simulink model "StarshotACS"  (R2017a)
settings: Solver=FixedStepAuto  StartTime=0.0  StopTime=6000  FixedStep=.1  MaxStep=4.0  MinStep=.001  RelTol=1e-6
undefined symbols (not defined in the file or in its folder): DiscIntNeverNeededParam, starshot
libraries: simulink x2, dspmathops x1
settings Model: Creator=armen  LastModifiedBy=armen
settings OptimizationCC: DefaultParameterBehavior=Inlined  UseDivisionForNetSlopeComputation=on  UseFloatMulNetSlope=on  InlineInvariantSignals=on  PassReuseOutputArgsAs=Individual arguments  ZeroExternalMemoryAtStartup=off  ZeroInternalMemoryAtStartup=off  NoFixptDivByZeroProtection=on  EfficientFloat2IntCast=on  LifeSpan=1
settings DebuggingCC: ParameterTunabilityLossMsg=error  FrameProcessingCompatibilityMsg=none
settings HardwareCC: ProdBitPerPointer=32  ProdBitPerSizeT=32  ProdBitPerPtrDiffT=32  ProdLargestAtomicInteger=Long  ProdLargestAtomicFloat=Double  ProdWordSize=32  ProdHWDeviceType=ARM Compatible->ARM Cortex
settings SFSimCC: MATLABDynamicMemAlloc=off
settings RTWCC: SystemTargetFile=ert.tlc  TLCOptions=-aAlwaysIncludeCustomSrc=1  GenCodeOnly=on  TemplateMakefile=ert_default_tmf  Description=Embedded Coder  GenerateReport=on  IncludeHyperlinkInReport=on  LaunchReport=on  TargetLang=C++  GenerateTraceInfo=on  GenerateTraceReport=on  GenerateTraceReportSl=on  GenerateTraceReportSf=on  GenerateTraceReportEml=on
settings CodeAppCC: ForceParamTrailComments=on  IgnoreCustomStorageClasses=off  OperatorAnnotations=on  SimulinkDataObjDesc=on  SFDataObjDesc=on  MATLABFcnDesc=on  CustomSymbolStrGlobalVar=rt$N$M  CustomSymbolStrType=$N$M  CustomSymbolStrFcn=$N$M$F  CustomSymbolStrMacro=$N$M  InsertBlockDesc=on  MATLABSourceComments=on
settings ERTTargetCC: TargetLangStandard=C++03 (ISO)  GenerateSampleERTMain=on  IncludeMdlTerminateFcn=off  CombineSignalStateStructs=on  SupportAbsoluteTime=off  MultiInstanceERTCode=on  CodeInterfacePackaging=C++ class  SupportComplex=off  SupportNonInlinedSFcns=on  InlinedParameterPlacement=NonHierarchical  RootIOFormat=Structure reference  ERTCustomFileTemplate=example_file_process.tlc  ERTFilePackagingFormat=CompactWithDataFile

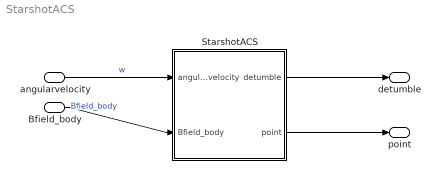
== system StarshotACS ==
  angularvelocity : Inport  OutDataTypeStr=double  PortDimensions=3  SampleTime=[0.10000000000000001 0]  Interpolate=off
  Bfield_body : Inport  Port=2  OutDataTypeStr=double  PortDimensions=3  SampleTime=[0.10000000000000001 0]  Interpolate=off
  StarshotACS : Subsystem  Tag=starshotsimv5  TreatAsAtomicUnit=on
      settings: RTWSystemCode=Inline
  detumble : Outport  OutDataTypeStr=double  PortDimensions=3  SampleTime=[0.10000000000000001 0]
  point : Outport  Port=2  OutDataTypeStr=double  PortDimensions=3  SampleTime=[0.10000000000000001 0]
  wires:
  angularvelocity/1 -> StarshotACS/1(angularvelocity)  "w"
  Bfield_body/1 -> StarshotACS/2(Bfield_body)  "Bfield_body"
  StarshotACS/1(detumble) -> detumble/1
  StarshotACS/2(point) -> point/1

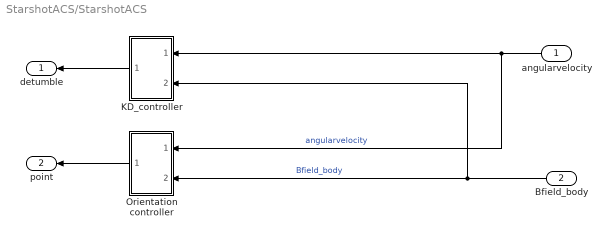
== system StarshotACS/StarshotACS ==
  angularvelocity : Inport
  Bfield_body : Inport  Port=2
  KD_controller : Subsystem
  Orientation controller : Subsystem
  detumble : Outport
  point : Outport  Port=2
  wires:
  angularvelocity/1 -> KD_controller/1(Omega), Orientation controller/1(Omega)  "angularvelocity"
  Bfield_body/1 -> Orientation controller/2(B(body)), KD_controller/2(B(body))  "Bfield_body"
  Orientation controller/1(Dipole) -> point/1
  KD_controller/1(Dipole) -> detumble/1

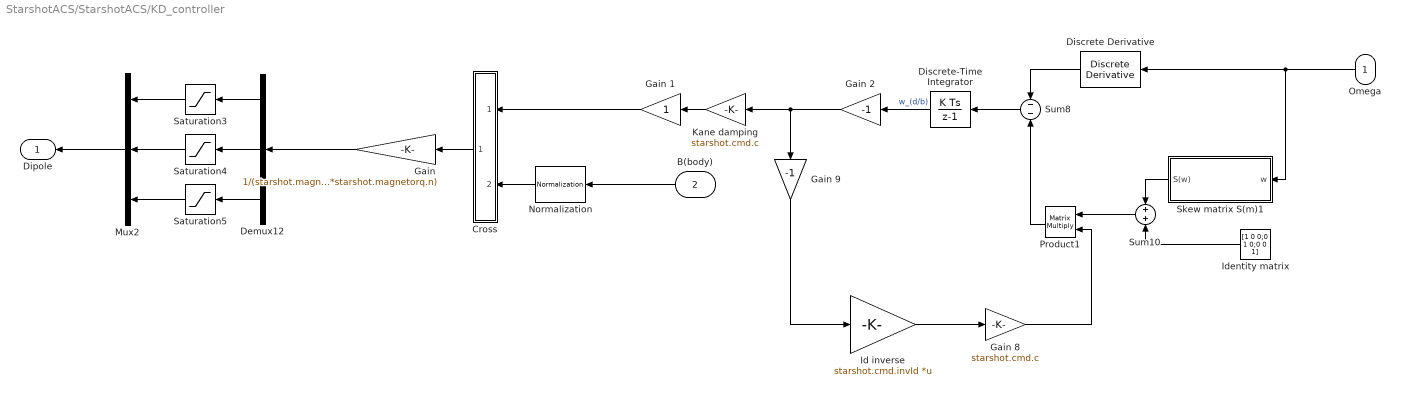
== system StarshotACS/StarshotACS/KD_controller ==
  Omega : Inport
  B(body) : Inport  Port=2
  Cross : Subsystem
  Demux12 : Demux  Outputs=3
  Discrete Derivative : simulink/Discrete/Discrete Derivative  gainval=1.0  ICPrevScaledInput=0.0  OutMin=[]  OutMax=[]  OutDataType=fixdt(1, 16)  OutScaling=2^-10  DoSatur=off
  Discrete-Time Integrator : DiscreteIntegrator  InitialCondition=starshot.cmd.wdb0  InitialConditionSetting=State (most efficient)  SampleTime=-1  ICPrevOutput=DiscIntNeverNeededParam  ICPrevScaledInput=DiscIntNeverNeededParam
  Gain : Gain  Gain=1/(starshot.magnetorq.A*starshot.magnetorq.n)
  Gain 1 : Gain  SaturateOnIntegerOverflow=on  OutDataTypeStr=Inherit: Same as input  ParamDataTypeStr=Inherit: Same as input
  Gain 2 : Gain  Gain=-1  SaturateOnIntegerOverflow=on  OutDataTypeStr=Inherit: Same as input  ParamDataTypeStr=Inherit: Same as input
  Gain 8 : Gain  Gain=starshot.cmd.c  SaturateOnIntegerOverflow=on  OutDataTypeStr=Inherit: Same as input  ParamDataTypeStr=Inherit: Same as input
  Gain 9 : Gain  Gain=-1  SaturateOnIntegerOverflow=on  OutDataTypeStr=Inherit: Same as input  ParamDataTypeStr=Inherit: Same as input
  Id inverse : Gain  Gain=starshot.cmd.invId  Multiplication=Matrix(K*u)  SaturateOnIntegerOverflow=on  OutDataTypeStr=Inherit: Same as input  ParamDataTypeStr=Inherit: Same as input
  Identity matrix : Constant  Value=[1 0 0;0 1 0;0 0 1]
  Kane damping : Gain  Gain=starshot.cmd.c  SaturateOnIntegerOverflow=on  OutDataTypeStr=Inherit: Same as input  ParamDataTypeStr=Inherit: Same as input
  Mux2 : Mux  Inputs=3
  Normalization : dspmathops/Normalization  NormType=Squared 2-norm  Bias=1e-10  NormOver=Each column  Dimension=1  outputDataTypeStr=Inherit: Same as product output  outputLastDataTypeStr=Inherit: Same as product output  outputMin=[]  outputMax=[]  accumDataTypeStr=Inherit: Same as product output  accumLastDataTypeStr=Inherit: Same as product output  roundingMode=Floor  overflowMode=off
      settings: SourceProductName=DSP System Toolbox
  Product1 : Product  Multiplication=Matrix(*)
  Saturation3 : Saturate  UpperLimit=starshot.magnetorq.m_max_x/(starshot.magnetorq.A*starshot.magnetorq.n)  LowerLimit=-starshot.magnetorq.m_max_x/(starshot.magnetorq.A*starshot.magnetorq.n)
  Saturation4 : Saturate  UpperLimit=starshot.magnetorq.m_max_y/(starshot.magnetorq.A*starshot.magnetorq.n)  LowerLimit=-starshot.magnetorq.m_max_y/(starshot.magnetorq.A*starshot.magnetorq.n)
  Saturation5 : Saturate  UpperLimit=starshot.magnetorq.m_max_z/(starshot.magnetorq.A*starshot.magnetorq.n)  LowerLimit=-starshot.magnetorq.m_max_z/(starshot.magnetorq.A*starshot.magnetorq.n)
  Skew matrix S(m)1 : Subsystem
  Sum10 : Sum  Inputs=+|+  SaturateOnIntegerOverflow=on  InputSameDT=on  OutDataTypeStr=Inherit: Same as first input
  Sum8 : Sum  Inputs=--
  Dipole : Outport
  wires:
  Mux2/1 -> Dipole/1
  Demux12/3 -> Saturation5/1
  Saturation4/1 -> Mux2/2
  Demux12/2 -> Saturation4/1
  Saturation5/1 -> Mux2/3
  Saturation3/1 -> Mux2/1
  Demux12/1 -> Saturation3/1
  Gain/1 -> Demux12/1
  Gain 1/1 -> Cross/1(A)
  Product1/1 -> Sum8/2
  Sum10/1 -> Product1/1
  Gain 9/1 -> Id inverse/1
  Identity matrix/1 -> Sum10/2
  Skew matrix S(m)1/1(S(w)) -> Sum10/1
  Id inverse/1 -> Gain 8/1
  Gain 8/1 -> Product1/2
  Sum8/1 -> Discrete-Time Integrator/1
  Discrete Derivative/1 -> Sum8/1
  Kane damping/1 -> Gain 1/1
  Normalization/1 -> Cross/2(B)
  Gain 2/1 -> Gain 9/1, Kane damping/1
  Cross/1(AxB) -> Gain/1
  B(body)/1 -> Normalization/1
  Omega/1 -> Skew matrix S(m)1/1(w), Discrete Derivative/1
  Discrete-Time Integrator/1 -> Gain 2/1  "w_(d/b)"

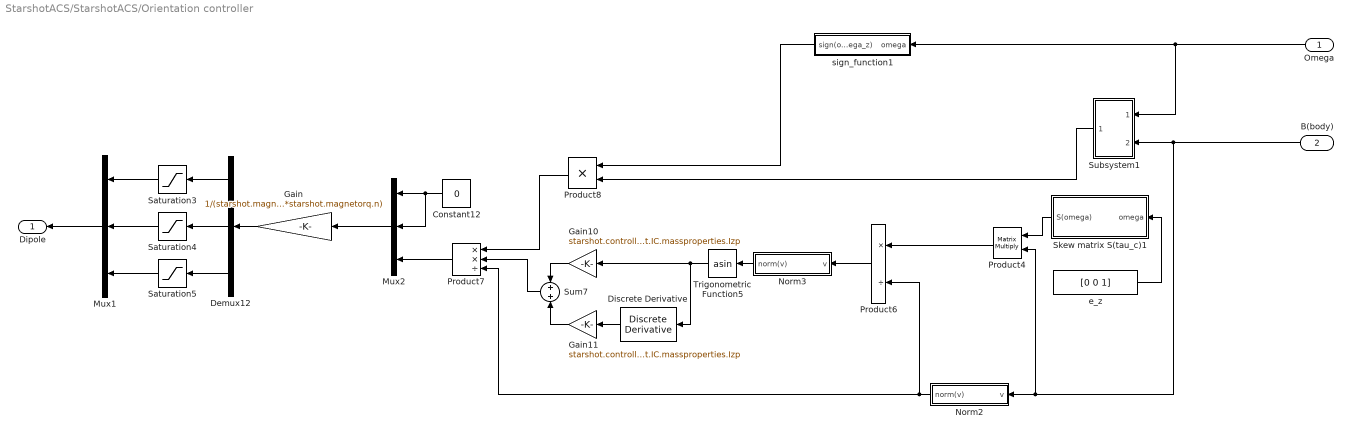
== system StarshotACS/StarshotACS/Orientation controller ==
  Omega : Inport
  B(body) : Inport  Port=2
  Constant12 : Constant  Value=0
  Demux12 : Demux  Outputs=3
  Discrete Derivative : simulink/Discrete/Discrete Derivative  gainval=1.0  ICPrevScaledInput=0.0  OutMin=[]  OutMax=[]  OutDataType=fixdt(1, 16)  OutScaling=2^-10  DoSatur=off
  Gain : Gain  Gain=1/(starshot.magnetorq.A*starshot.magnetorq.n)
  Gain10 : Gain  Gain=starshot.controller.Kp*starshot.IC.massproperties.Izp
  Gain11 : Gain  Gain=starshot.controller.Kd*starshot.IC.massproperties.Izp
  Mux1 : Mux  Inputs=3
  Mux2 : Mux  Inputs=3
  Norm2 : Subsystem
  Norm3 : Subsystem
  Product4 : Product  Multiplication=Matrix(*)
  Product6 : Product  Inputs=*/
  Product7 : Product  Inputs=**/
  Product8 : Product  Inputs=**
  Saturation3 : Saturate  UpperLimit=starshot.magnetorq.m_max_x/(starshot.magnetorq.A*starshot.magnetorq.n)  LowerLimit=-starshot.magnetorq.m_max_x/(starshot.magnetorq.A*starshot.magnetorq.n)
  Saturation4 : Saturate  UpperLimit=starshot.magnetorq.m_max_y/(starshot.magnetorq.A*starshot.magnetorq.n)  LowerLimit=-starshot.magnetorq.m_max_y/(starshot.magnetorq.A*starshot.magnetorq.n)
  Saturation5 : Saturate  UpperLimit=starshot.magnetorq.m_max_z/(starshot.magnetorq.A*starshot.magnetorq.n)  LowerLimit=-starshot.magnetorq.m_max_z/(starshot.magnetorq.A*starshot.magnetorq.n)
  Skew matrix S(tau_c)1 : Subsystem
  Subsystem1 : Subsystem
  Sum7 : Sum  Inputs=+|+
  Trigonometric Function5 : Trigonometry  Operator=asin
  e_z : Constant  Value=[0 0 1]
  sign_function1 : Subsystem
  Dipole : Outport
  wires:
  Mux1/1 -> Dipole/1
  Demux12/3 -> Saturation5/1
  Saturation4/1 -> Mux1/2
  Demux12/2 -> Saturation4/1
  Saturation5/1 -> Mux1/3
  Saturation3/1 -> Mux1/1
  Demux12/1 -> Saturation3/1
  Gain/1 -> Demux12/1
  Omega/1 -> sign_function1/1(omega), Subsystem1/1(omega)
  Subsystem1/1(sign(cos)) -> Product8/2
  sign_function1/1(sign(omega_z)) -> Product8/1
  B(body)/1 -> Subsystem1/2(B(body)), Norm2/1(v), Product4/2
  Gain11/1 -> Sum7/2
  Product8/1 -> Product7/1
  Product6/1 -> Norm3/1(v)
  Gain10/1 -> Sum7/1
  Norm2/1(norm(v)) -> Product6/2, Product7/3
  Discrete Derivative/1 -> Gain11/1
  Skew matrix S(tau_c)1/1(S(omega)) -> Product4/1
  Constant12/1 -> Mux2/1, Mux2/2
  Product7/1 -> Mux2/3
  e_z/1 -> Skew matrix S(tau_c)1/1(omega)
  Norm3/1(norm(v)) -> Trigonometric Function5/1
  Trigonometric Function5/1 -> Discrete Derivative/1, Gain10/1
  Sum7/1 -> Product7/2
  Mux2/1 -> Gain/1
  Product4/1 -> Product6/1

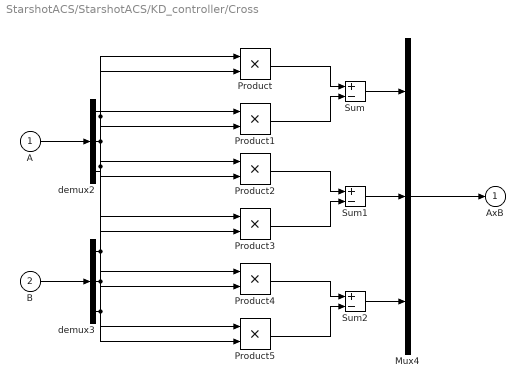
== system StarshotACS/StarshotACS/KD_controller/Cross ==
  A : Inport
  B : Inport  Port=2
  Mux4 : Mux  Inputs=3
  Product{,1..5} (6 alike) : Product  SaturateOnIntegerOverflow=on  InputSameDT=on  OutDataTypeStr=Inherit: Same as first input
  Sum : Sum  Inputs=+-  SaturateOnIntegerOverflow=on  InputSameDT=on  OutDataTypeStr=Inherit: Same as first input
  Sum1 : Sum  Inputs=+-  SaturateOnIntegerOverflow=on  InputSameDT=on  OutDataTypeStr=Inherit: Same as first input
  Sum2 : Sum  Inputs=+-  SaturateOnIntegerOverflow=on  InputSameDT=on  OutDataTypeStr=Inherit: Same as first input
  demux2 : Demux  Outputs=3
  demux3 : Demux  Outputs=3
  AxB : Outport  InitialOutput=0
  wires:
  Mux4/1 -> AxB/1
  Sum2/1 -> Mux4/3
  Sum1/1 -> Mux4/2
  Sum/1 -> Mux4/1
  Product5/1 -> Sum2/2
  Product4/1 -> Sum2/1
  Product3/1 -> Sum1/2
  Product2/1 -> Sum1/1
  Product1/1 -> Sum/2
  Product/1 -> Sum/1
  demux3/1 -> Product5/2, Product2/2
  demux2/2 -> Product5/1, Product/1
  demux3/2 -> Product4/2, Product1/2
  demux2/1 -> Product4/1, Product3/1
  demux3/3 -> Product3/2, Product/2
  demux2/3 -> Product2/1, Product1/1
  B/1 -> demux3/1
  A/1 -> demux2/1

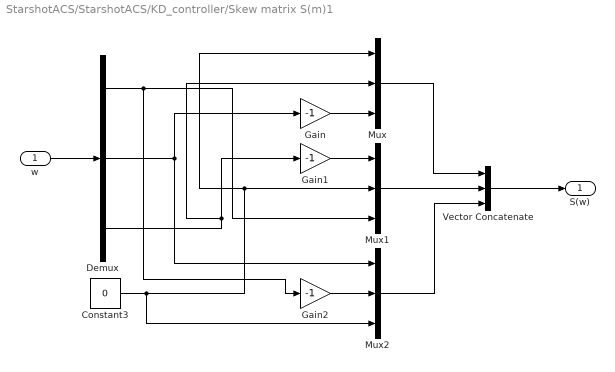
== system StarshotACS/StarshotACS/KD_controller/Skew matrix S(m)1 ==
  w : Inport
  Constant3 : Constant  Value=0
  Demux : Demux  Outputs=3
  Gain : Gain  Gain=-1
  Gain1 : Gain  Gain=-1
  Gain2 : Gain  Gain=-1
  Mux : Mux  Inputs=3
  Mux1 : Mux  Inputs=3
  Mux2 : Mux  Inputs=3
  Vector Concatenate : Concatenate  NumInputs=3  Mode=Multidimensional array  ConcatenateDimension=2
  S(w) : Outport
  wires:
  Gain1/1 -> Mux1/1
  Mux2/1 -> Vector Concatenate/3
  Mux/1 -> Vector Concatenate/1
  Vector Concatenate/1 -> S(w)/1
  Constant3/1 -> Mux1/2, Mux/1, Mux2/3
  w/1 -> Demux/1
  Mux1/1 -> Vector Concatenate/2
  Demux/1 -> Gain2/1, Mux1/3
  Gain2/1 -> Mux2/2
  Demux/3 -> Mux/2, Gain1/1
  Demux/2 -> Gain/1, Mux2/1
  Gain/1 -> Mux/3

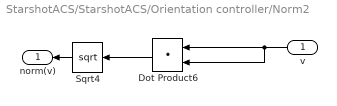
== system StarshotACS/StarshotACS/Orientation controller/Norm2 ==
  v : Inport
  Dot Product6 : DotProduct  InputSameDT=on  OutDataTypeStr=Inherit: Inherit via internal rule
  Sqrt4 : Sqrt  SaturateOnIntegerOverflow=on
  norm(v) : Outport
  wires:
  Sqrt4/1 -> norm(v)/1
  Dot Product6/1 -> Sqrt4/1
  v/1 -> Dot Product6/2, Dot Product6/1

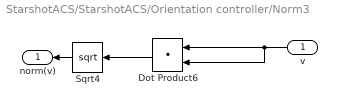
== system StarshotACS/StarshotACS/Orientation controller/Norm3 ==
  v : Inport
  Dot Product6 : DotProduct  InputSameDT=on  OutDataTypeStr=Inherit: Inherit via internal rule
  Sqrt4 : Sqrt  SaturateOnIntegerOverflow=on
  norm(v) : Outport
  wires:
  Sqrt4/1 -> norm(v)/1
  Dot Product6/1 -> Sqrt4/1
  v/1 -> Dot Product6/2, Dot Product6/1

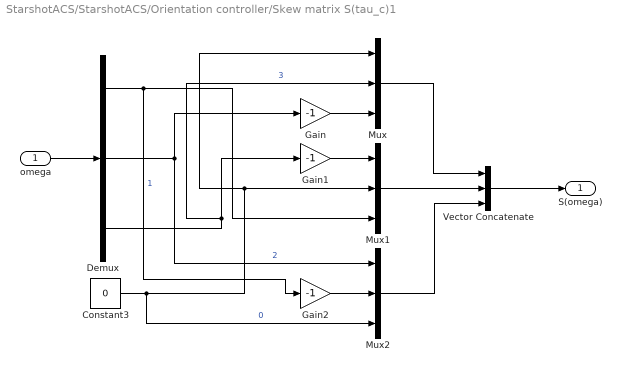
== system StarshotACS/StarshotACS/Orientation controller/Skew matrix S(tau_c)1 ==
  omega : Inport
  Constant3 : Constant  Value=0
  Demux : Demux  Outputs=3
  Gain : Gain  Gain=-1
  Gain1 : Gain  Gain=-1
  Gain2 : Gain  Gain=-1
  Mux : Mux  Inputs=3
  Mux1 : Mux  Inputs=3
  Mux2 : Mux  Inputs=3
  Vector Concatenate : Concatenate  NumInputs=3  Mode=Multidimensional array  ConcatenateDimension=2
  S(omega) : Outport
  wires:
  Gain1/1 -> Mux1/1
  Mux2/1 -> Vector Concatenate/3
  Mux/1 -> Vector Concatenate/1
  Vector Concatenate/1 -> S(omega)/1
  Constant3/1 -> Mux1/2, Mux/1, Mux2/3  "0"
  omega/1 -> Demux/1
  Mux1/1 -> Vector Concatenate/2
  Demux/1 -> Gain2/1, Mux1/3  "1"
  Gain2/1 -> Mux2/2
  Demux/3 -> Mux/2, Gain1/1  "3"
  Demux/2 -> Gain/1, Mux2/1  "2"
  Gain/1 -> Mux/3

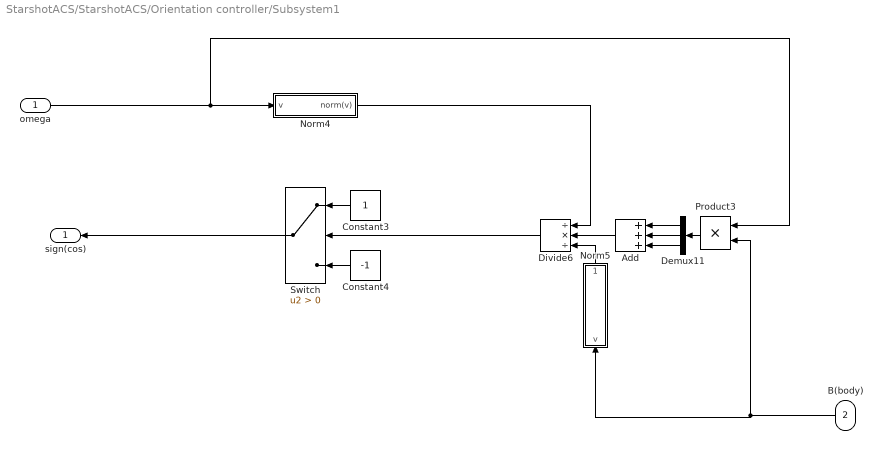
== system StarshotACS/StarshotACS/Orientation controller/Subsystem1 ==
  omega : Inport
  B(body) : Inport  Port=2
  Add : Sum  Inputs=3
  Constant3 : Constant
  Constant4 : Constant  Value=-1
  Demux11 : Demux  Outputs=3
  Divide6 : Product  Inputs=/*/
  Norm4 : Subsystem
  Norm5 : Subsystem
  Product3 : Product
  Switch : Switch  Criteria=u2 > Threshold  ZeroCross=off
  sign(cos) : Outport
  wires:
  omega/1 -> Norm4/1(v), Product3/1
  B(body)/1 -> Product3/2, Norm5/1(v)
  Demux11/2 -> Add/2
  Demux11/1 -> Add/1
  Product3/1 -> Demux11/1
  Norm5/1(norm(v)) -> Divide6/3
  Divide6/1 -> Switch/2
  Norm4/1(norm(v)) -> Divide6/1
  Demux11/3 -> Add/3
  Constant3/1 -> Switch/1
  Add/1 -> Divide6/2
  Constant4/1 -> Switch/3
  Switch/1 -> sign(cos)/1

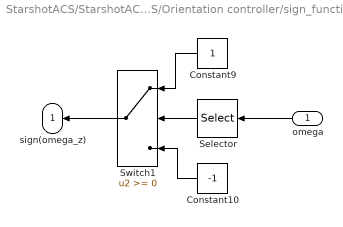
== system StarshotACS/StarshotACS/Orientation controller/sign_function1 ==
  omega : Inport
  Constant10 : Constant  Value=-1
  Constant9 : Constant
  Selector : Selector  InputPortWidth=3  IndexOptions=Index vector (dialog)  Indices=[3]  OutputSizes=1
  Switch1 : Switch  ZeroCross=off
  sign(omega_z) : Outport
  wires:
  omega/1 -> Selector/1
  Selector/1 -> Switch1/2
  Switch1/1 -> sign(omega_z)/1
  Constant10/1 -> Switch1/3
  Constant9/1 -> Switch1/1

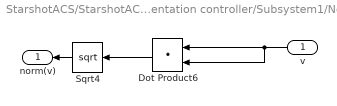
== system StarshotACS/StarshotACS/Orientation controller/Subsystem1/Norm4 ==
  v : Inport
  Dot Product6 : DotProduct  InputSameDT=on  OutDataTypeStr=Inherit: Inherit via internal rule
  Sqrt4 : Sqrt  SaturateOnIntegerOverflow=on
  norm(v) : Outport
  wires:
  Sqrt4/1 -> norm(v)/1
  Dot Product6/1 -> Sqrt4/1
  v/1 -> Dot Product6/2, Dot Product6/1

== system StarshotACS/StarshotACS/Orientation controller/Subsystem1/Norm5 ==
  v : Inport
  Dot Product6 : DotProduct  InputSameDT=on  OutDataTypeStr=Inherit: Inherit via internal rule
  Sqrt4 : Sqrt  SaturateOnIntegerOverflow=on
  norm(v) : Outport
  wires:
  Sqrt4/1 -> norm(v)/1
  Dot Product6/1 -> Sqrt4/1
  v/1 -> Dot Product6/2, Dot Product6/1
